simulink model "EX005_FCHEVwithCooling"  (R2023a)
settings: Solver=ode23tb  StartTime=0.0  StopTime=20e3  MaxStep=1e-1  RelTol=1e-4
libraries: component_lib x35, slpidlib x3, simulink x1
settings Model: Creator=maxjo65  LastModifiedBy=maxjo
settings OptimizationCC: ReuseModelBlockBuffer=off
settings DebuggingCC: UnconnectedInputMsg=warning  UnconnectedOutputMsg=warning  UnconnectedLineMsg=warning
settings ModelReferenceCC: EnableRefExpFcnMdlSchedulingChecks=on
settings RTWCC: DLArmComputeVersion=19.05

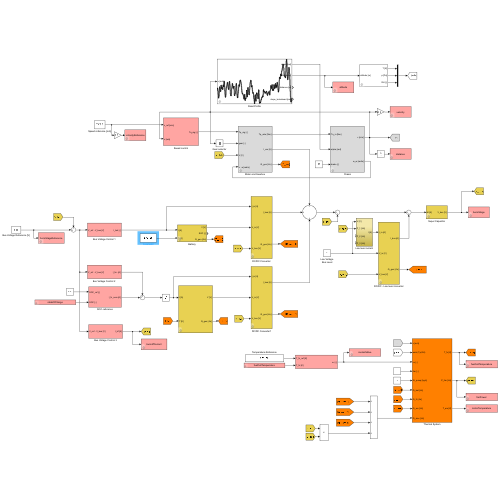
[thumbnail: Simulink's stored preview of the top-level diagram]
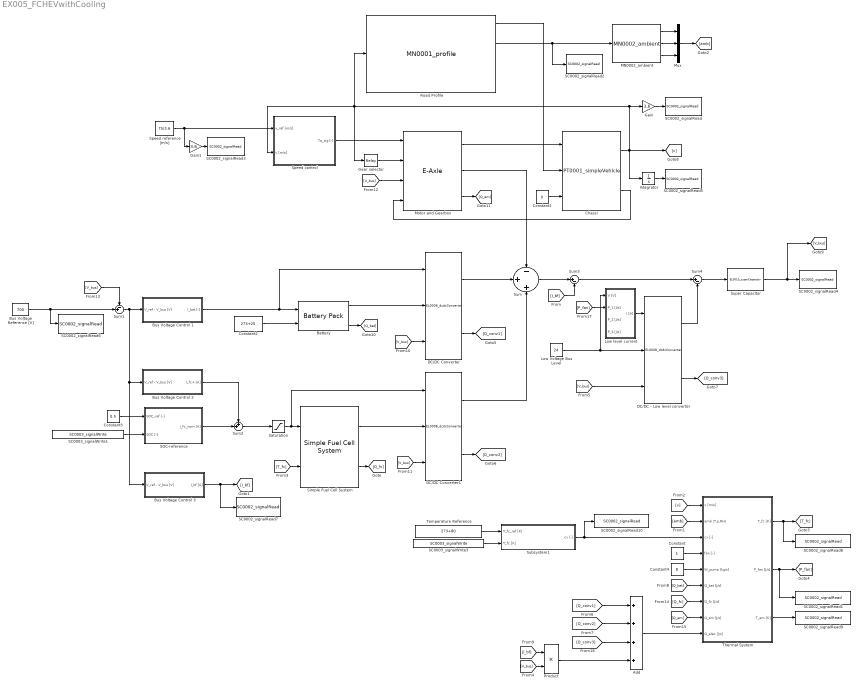
== system EX005_FCHEVwithCooling ==
  Add : Sum  Inputs=++++
  Battery : component_lib/Battery Pack  SOC_0=0.5  Nx=120  Ny=180
  Bus Voltage Control 1 : Subsystem
  "Bus Voltage Control 2 " : Subsystem
  Bus Voltage Control 3 : Subsystem
  Bus Voltage Reference [V] : Constant  Value=700
  Chassi : component_lib/Powertrain/PT0001_simpleVehicle  m=40e3  r_w=0.5  A_f=10  C_d=0.5  rho_air=1.225  c_r0=0.0060  c_r1=2.3e-7  gain=600  v0=75/3.6  x0=0
  Constant : Constant
  Constant1 : Constant  Value=0
  Constant2 : Constant  Value=273+25
  Constant3 : Constant  Value=0.5
  Constant4 : Constant  Value=8
  DC/DC - Low level converter : component_lib/Electrochemistry/EL0008_dcdcConverter  eta_up=0.99  eta_down=0.99
  DC/DC Converter : component_lib/Electrochemistry/EL0008_dcdcConverter  eta_up=0.99  eta_down=0.99
  DC/DC Converter1 : component_lib/Electrochemistry/EL0008_dcdcConverter  eta_up=0.99  eta_down=0.99
  Gain : Gain  Gain=3.6
  Gain1 : Gain  Gain=3.6
  Gear selector : Relay  OnSwitchValue=22  OffSwitchValue=21.5  OnOutputValue=4  OffOutputValue=3
  Integrator : Integrator
  Low Voltage Bus Level : Constant  Value=24
  Low level current : Subsystem
  MN0002_ambient : component_lib/Mission/MN0002_ambient  p_0=1.01e5  T_0=273 + 20  RH_0=0.05
  Motor and Gearbox : component_lib/E-Axle  n=3  V_nom=700
  Mux : Mux  Inputs=3
  Product : Product
  Road Profile : component_lib/Mission/MN0001_profile  profile=Sodertalje_Norrkoping.mat  x0=0  N_lookahead=100
  SC0002_signalRead : component_lib/Data & Control/SC0002_signalRead  SigName=velocity
  SC0002_signalRead1 : component_lib/Data & Control/SC0002_signalRead  SigName=fanPower
  SC0002_signalRead10 : component_lib/Data & Control/SC0002_signalRead  SigName=coolantValve
  SC0002_signalRead2 : component_lib/Data & Control/SC0002_signalRead  SigName=altitude
  SC0002_signalRead3 : component_lib/Data & Control/SC0002_signalRead  SigName=velocityReference
  SC0002_signalRead4 : component_lib/Data & Control/SC0002_signalRead  SigName=busVoltage
  SC0002_signalRead5 : component_lib/Data & Control/SC0002_signalRead  SigName=distance
  SC0002_signalRead6 : component_lib/Data & Control/SC0002_signalRead  SigName=busVoltageReference
  SC0002_signalRead7 : component_lib/Data & Control/SC0002_signalRead  SigName=burnoffCurrent
  SC0002_signalRead8 : component_lib/Data & Control/SC0002_signalRead  SigName=fuelCellTemperature
  SC0002_signalRead9 : component_lib/Data & Control/SC0002_signalRead  SigName=motorTemperature
  SC0003_signalWrite1 : component_lib/Data & Control/SC0003_signalWrite  SigName=stateOfCharge
  SC0003_signalWrite3 : component_lib/Data & Control/SC0003_signalWrite  SigName=fuelCellTemperature
  SOC-reference : Subsystem
  Saturation : Saturate  UpperLimit=600  LowerLimit=20
  Simple Fuel Cell System : component_lib/Simple Fuel Cell System  n_st=2  n=375
  Speed control : Subsystem
  Speed reference [m/s] : Constant  Value=75/3.6
  Subsystem1 : Subsystem
  Sum : Sum  Inputs=-++
  Sum1 : Sum  Inputs=-+|
  Sum2 : Sum  Inputs=++|
  Sum3 : Sum  Inputs=|+-
  Sum4 : Sum  Inputs=|+-
  Super Capacitor : component_lib/Electrochemistry/EL0010_superCapacitor  C=1  V_bus0=700
  Temperature Reference : Constant  Value=273+80
  Thermal System : Subsystem
  wires:
  Motor and Gearbox/1 -> Chassi/1
  Chassi/2 -> Motor and Gearbox/4
  Road Profile/1 -> Chassi/2
  Speed reference [m/s]/1 -> Gain1/1, Speed control/1(v_ref [m/s])
  Gear selector/1 -> Motor and Gearbox/2
  Integrator/1 -> SC0002_signalRead5/1
  Gain/1 -> SC0002_signalRead/1
  Road Profile/2 -> MN0002_ambient/1, SC0002_signalRead2/1
  Gain1/1 -> SC0002_signalRead3/1
  Super Capacitor/1 -> SC0002_signalRead4/1, [V_bus]
  Constant1/1 -> Chassi/3
  Battery/1 -> DC/DC Converter/2
  DC/DC Converter/1 -> Sum/2
  Motor and Gearbox/2 -> Sum/1
  Bus Voltage Control 1/1(I_bat [-]) -> Battery/1, DC/DC Converter/1
  DC/DC Converter1/1 -> Sum/3
  Bus Voltage Reference [V]/1 -> Sum1/2, SC0002_signalRead6/1
  Constant3/1 -> SOC-reference/1(SOC_ref [-])
  SC0003_signalWrite1/1 -> SOC-reference/2(SOC [-])
  Sum1/1 -> Bus Voltage Control 3/1(V_ref - V_bus [V]), "Bus Voltage Control 2 "/1(V_ref - V_bus [V]), Bus Voltage Control 1/1(V_ref - V_bus [V])
  "Bus Voltage Control 2 "/1(I_fc+ [A]) -> Sum2/1
  SOC-reference/1(I_fc_nom [A]) -> Sum2/2
  Sum/1 -> Sum3/1
  Bus Voltage Control 3/1(I_bf [A]) -> SC0002_signalRead7/1, [I_bf]
  [I_bf] -> Sum3/2
  MN0002_ambient/3 -> Mux/3
  MN0002_ambient/1 -> Mux/1
  MN0002_ambient/2 -> Mux/2
  Mux/1 -> [amb]
  Simple Fuel Cell System/1 -> DC/DC Converter1/2
  Saturation/1 -> Simple Fuel Cell System/1, DC/DC Converter1/1
  Sum3/1 -> Sum4/1
  Thermal System/2(P_fan [J/s]) -> [P_fan], SC0002_signalRead1/1
  Constant4/1 -> Thermal System/5(W_pump [kg/s])
  [Q_em] -> Thermal System/8(Q_em [J/s])
  Thermal System/1(T_fc [K]) -> [T_fc], SC0002_signalRead8/1
  [Q_bat] -> Thermal System/6(Q_bat [J/s])
  Subsystem1/1(cv [-]) -> Thermal System/3(cv [-]), SC0002_signalRead10/1
  [v] -> Thermal System/1(v [m/s])
  Constant/1 -> Thermal System/4(fan [-])
  Thermal System/3(T_em [K]) -> SC0002_signalRead9/1
  [Q_fc] -> Thermal System/7(Q_fc [J/s])
  [amb] -> Thermal System/2(amb (T,p,RH))
  Low Voltage Bus Level/1 -> DC/DC - Low level converter/2, Low level current/1(V [V])
  DC/DC - Low level converter/1 -> Sum4/2
  Sum4/1 -> Super Capacitor/1
  Add/1 -> Thermal System/9(Q_elec [J/s])
  [Q_conv1] -> Add/1
  [Q_conv2] -> Add/2
  [Q_conv3] -> Add/3
  DC/DC Converter/2 -> [Q_conv1]
  DC/DC Converter1/2 -> [Q_conv2]
  DC/DC - Low level converter/2 -> [Q_conv3]
  [V_bus] -> Motor and Gearbox/3
  [V_bus] -> Sum1/1
  Battery/3 -> [Q_bat]
  Simple Fuel Cell System/2 -> [Q_fc]
  [I_bf] -> Product/1
  [V_bus] -> Product/2
  Product/1 -> Add/4
  Motor and Gearbox/3 -> [Q_em]
  Temperature Reference/1 -> Subsystem1/1(T_fc_ref [K])
  Chassi/1 -> Integrator/1, [v], Gain/1, Road Profile/1, Speed control/2(v [m/s]), Gear selector/1
  SC0003_signalWrite3/1 -> Subsystem1/2(T_fc [K])
  [P_fan] -> Low level current/2(P_1 [J/s])
  [T_fc] -> Simple Fuel Cell System/2
  Speed control/1(Tq_sig [-]) -> Motor and Gearbox/1
  Sum2/1 -> Saturation/1
  [V_bus] -> DC/DC Converter/3
  [V_bus] -> DC/DC Converter1/3
  Constant2/1 -> Battery/2
  Low level current/1(I [A]) -> DC/DC - Low level converter/1
  [V_bus] -> DC/DC - Low level converter/3

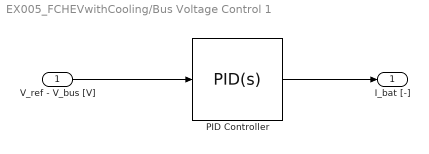
== system EX005_FCHEVwithCooling/Bus Voltage Control 1 ==
  V_ref - V_bus [V] : Inport
  PID Controller : slpidlib/PID Controller  Controller=PID  Form=Parallel  TimeDomain=Continuous-time  UseExternalTs=off  SampleTime=-1  IntegratorMethod=Forward Euler  FilterMethod=Forward Euler  ControllerParametersSource=internal  P=1e2  I=1  UseKiTs=off  D=0  N=100  UseFilter=on  TunerSelectOption=Transfer Function Based (PID Tuner App)  ZeroCross=off  InitialConditionSource=internal  InitialConditionForIntegrator=0  InitialConditionForFilter=0  DifferentiatorICPrevScaledInput=0  ExternalReset=none  TrackingMode=off  Kt=1  LimitOutput=on  SatLimitsSource=internal  UpperSaturationLimit=350  LowerSaturationLimit=-350  LinearizeAsGain=on  AntiWindupMode=clamping  Kb=1  LimitIntegrator=off  UpperIntegratorSaturationLimit=inf  LowerIntegratorSaturationLimit=-inf  POutMin=[]  POutMax=[]  IOutMin=[]  IOutMax=[]  DOutMin=[]  DOutMax=[]  NOutMin=[]  NOutMax=[]  SumOutMin=[]  SumOutMax=[]  SaturationOutMin=[]  SaturationOutMax=[]  PParamMin=[]  PParamMax=[]  IParamMin=[]  IParamMax=[]  DParamMin=[]  DParamMax=[]  NParamMin=[]  NParamMax=[]  KbParamMin=[]  KbParamMax=[]  KtParamMin=[]  KtParamMax=[]  KbOutMin=[]  KbOutMax=[]  KtOutMin=[]  KtOutMax=[]  IntegratorOutMin=[]  IntegratorOutMax=[]  FilterOutMin=[]  FilterOutMax=[]  SumI1OutMin=[]  SumI1OutMax=[]  SumI2OutMin=[]  SumI2OutMax=[]  SumI3OutMin=[]  SumI3OutMax=[]  SumI4OutMin=[]  SumI4OutMax=[]  SumDOutMin=[]  SumDOutMax=[]  DifferentiatorOutMin=[]  DifferentiatorOutMax=[]  FilterDiffOutCoefMin=[]  FilterDiffOutCoefMax=[]  ReciprocalOutMin=[]  ReciprocalOutMax=[]  SumDenOutMin=[]  SumDenOutMax=[]  SumNumOutMin=[]  SumNumOutMax=[]  DivideOutMin=[]  DivideOutMax=[]  UdiffTsProdOutMin=[]  UdiffTsProdOutMax=[]  NTsProdOutMin=[]  NTsProdOutMax=[]  UintegralTsProdOutMin=[]  UintegralTsProdOutMax=[]  UngainTsProdOutMin=[]  UngainTsProdOutMax=[]  ClampingZeroOutDataTypeStr=Inherit: Inherit via back propagation  ClampingZeroOutMin=[]  ClampingZeroOutMax=[]  FilterDenConstantOutDataTypeStr=Inherit: Inherit via back propagation  FilterDenConstantOutMin=[]  FilterDenConstantOutMax=[]  PCopyOutDataTypeStr=Inherit: Inherit via back propagation  PCopyOutMin=[]  PCopyOutMax=[]  NCopyOutDataTypeStr=Inherit: Inherit via back propagation  NCopyOutMin=[]  NCopyOutMax=[]  IntegratorContinuousStateAttributes=''  IntegratorStateMustResolveToSignalObject=off  IntegratorRTWStateStorageClass=Auto  FilterContinuousStateAttributes=''  FilterStateMustResolveToSignalObject=off  FilterRTWStateStorageClass=Auto  ParallelPVariant=InternalParameters  IdealPVariant=Disabled  IVariant=InternalParameters  DVariant=InternalParameters  IntegratorVariant=Continuous  SatVariant=Enabled  AWVariant=ContClampingParallel  PCopyVariant=Disabled  TRVariant=Disabled  FdbkBlocksVariant=Forward  IdealPFdbkVariant=Disabled  SatFdbkVariant=Disabled  DerivativeFilterVariant=ContFilter  NVariant=InternalParameters  NCopyVariant=Disabled  FilterICVariant=InternalICsFilter  IntegratorICVariant=InternalICs  ExternalResetVariant=Disabled  TRSumVariant=Passthrough  SumFdbkVariant=Disabled  SumVariant=Sum_PID  TsampFilterVariant=InternalTs  TsampNgainVariant=Passthrough  TsampIntegralVariant=Disabled_SignalSpec  ExternalSaturationOutDataTypeStr=Inherit: Same as second input
  I_bat [-] : Outport
  wires:
  PID Controller/1 -> I_bat [-]/1
  V_ref - V_bus [V]/1 -> PID Controller/1

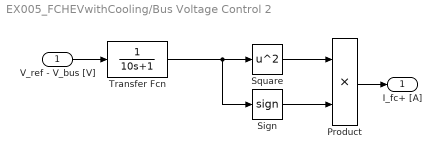
== system EX005_FCHEVwithCooling/Bus Voltage Control 2  ==
  V_ref - V_bus [V] : Inport
  Product : Product
  Sign : Signum
  Square : Math  Operator=square
  Transfer Fcn : TransferFcn  Denominator=[10 1]
  I_fc+ [A] : Outport
  wires:
  Sign/1 -> Product/2
  Transfer Fcn/1 -> Sign/1, Square/1
  Square/1 -> Product/1
  V_ref - V_bus [V]/1 -> Transfer Fcn/1
  Product/1 -> I_fc+ [A]/1

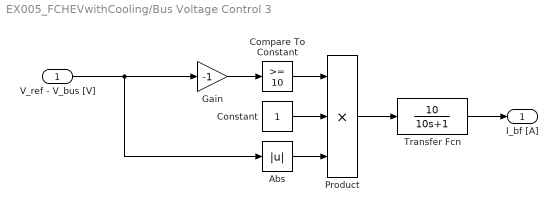
== system EX005_FCHEVwithCooling/Bus Voltage Control 3 ==
  V_ref - V_bus [V] : Inport
  Abs : Abs  SaturateOnIntegerOverflow=off
  Compare To Constant : simulink/Logic and Bit Operations/Compare To Constant  relop=>=  const=10  OutDataTypeStr=boolean
  Constant : Constant
  Gain : Gain  Gain=-1
  Product : Product  Inputs=3
  Transfer Fcn : TransferFcn  Numerator=[10]  Denominator=[10 1]
  I_bf [A] : Outport
  wires:
  Gain/1 -> Compare To Constant/1
  Transfer Fcn/1 -> I_bf [A]/1
  Compare To Constant/1 -> Product/1
  Product/1 -> Transfer Fcn/1
  V_ref - V_bus [V]/1 -> Abs/1, Gain/1
  Abs/1 -> Product/3
  Constant/1 -> Product/2

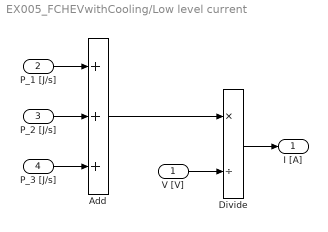
== system EX005_FCHEVwithCooling/Low level current ==
  V [V] : Inport
  P_1 [J/s] : Inport  Port=2
  P_2 [J/s] : Inport  Port=3
  P_3 [J/s] : Inport  Port=4
  Add : Sum  Inputs=+++
  Divide : Product  Inputs=*/
  I [A] : Outport
  wires:
  Add/1 -> Divide/1
  P_1 [J/s]/1 -> Add/1
  V [V]/1 -> Divide/2
  P_3 [J/s]/1 -> Add/3
  P_2 [J/s]/1 -> Add/2
  Divide/1 -> I [A]/1

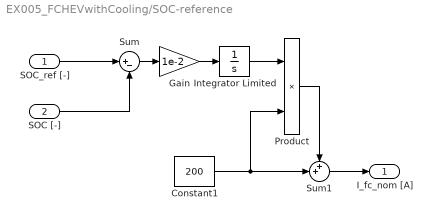
== system EX005_FCHEVwithCooling/SOC-reference ==
  SOC_ref [-] : Inport
  SOC [-] : Inport  Port=2
  Constant1 : Constant  Value=200
  Gain : Gain  Gain=1e-2
  Integrator Limited : Integrator  LimitOutput=on  UpperSaturationLimit=1  LowerSaturationLimit=-1
  Product : Product
  Sum : Sum  Inputs=|+-
  Sum1 : Sum  Inputs=++|
  I_fc_nom [A] : Outport
  wires:
  Product/1 -> Sum1/1
  Integrator Limited/1 -> Product/1
  Sum1/1 -> I_fc_nom [A]/1
  Constant1/1 -> Sum1/2, Product/2
  Sum/1 -> Gain/1
  SOC [-]/1 -> Sum/2
  Gain/1 -> Integrator Limited/1
  SOC_ref [-]/1 -> Sum/1

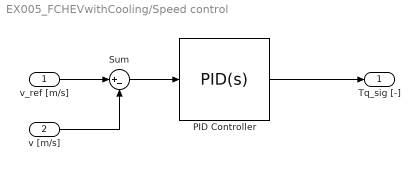
== system EX005_FCHEVwithCooling/Speed control ==
  v_ref [m/s] : Inport
  v [m/s] : Inport  Port=2
  PID Controller : slpidlib/PID Controller  Controller=PID  Form=Parallel  TimeDomain=Continuous-time  UseExternalTs=off  SampleTime=-1  IntegratorMethod=Forward Euler  FilterMethod=Forward Euler  ControllerParametersSource=internal  P=10  I=1e-1  UseKiTs=off  D=0  N=100  UseFilter=on  TunerSelectOption=Transfer Function Based (PID Tuner App)  ZeroCross=off  InitialConditionSource=internal  InitialConditionForIntegrator=0  InitialConditionForFilter=0  DifferentiatorICPrevScaledInput=0  ExternalReset=none  TrackingMode=off  Kt=1  LimitOutput=on  SatLimitsSource=internal  UpperSaturationLimit=1  LowerSaturationLimit=-1  LinearizeAsGain=on  AntiWindupMode=clamping  Kb=1  LimitIntegrator=off  UpperIntegratorSaturationLimit=inf  LowerIntegratorSaturationLimit=-inf  POutMin=[]  POutMax=[]  IOutMin=[]  IOutMax=[]  DOutMin=[]  DOutMax=[]  NOutMin=[]  NOutMax=[]  SumOutMin=[]  SumOutMax=[]  SaturationOutMin=[]  SaturationOutMax=[]  PParamMin=[]  PParamMax=[]  IParamMin=[]  IParamMax=[]  DParamMin=[]  DParamMax=[]  NParamMin=[]  NParamMax=[]  KbParamMin=[]  KbParamMax=[]  KtParamMin=[]  KtParamMax=[]  KbOutMin=[]  KbOutMax=[]  KtOutMin=[]  KtOutMax=[]  IntegratorOutMin=[]  IntegratorOutMax=[]  FilterOutMin=[]  FilterOutMax=[]  SumI1OutMin=[]  SumI1OutMax=[]  SumI2OutMin=[]  SumI2OutMax=[]  SumI3OutMin=[]  SumI3OutMax=[]  SumI4OutMin=[]  SumI4OutMax=[]  SumDOutMin=[]  SumDOutMax=[]  DifferentiatorOutMin=[]  DifferentiatorOutMax=[]  FilterDiffOutCoefMin=[]  FilterDiffOutCoefMax=[]  ReciprocalOutMin=[]  ReciprocalOutMax=[]  SumDenOutMin=[]  SumDenOutMax=[]  SumNumOutMin=[]  SumNumOutMax=[]  DivideOutMin=[]  DivideOutMax=[]  UdiffTsProdOutMin=[]  UdiffTsProdOutMax=[]  NTsProdOutMin=[]  NTsProdOutMax=[]  UintegralTsProdOutMin=[]  UintegralTsProdOutMax=[]  UngainTsProdOutMin=[]  UngainTsProdOutMax=[]  ClampingZeroOutDataTypeStr=Inherit: Inherit via back propagation  ClampingZeroOutMin=[]  ClampingZeroOutMax=[]  FilterDenConstantOutDataTypeStr=Inherit: Inherit via back propagation  FilterDenConstantOutMin=[]  FilterDenConstantOutMax=[]  PCopyOutDataTypeStr=Inherit: Inherit via back propagation  PCopyOutMin=[]  PCopyOutMax=[]  NCopyOutDataTypeStr=Inherit: Inherit via back propagation  NCopyOutMin=[]  NCopyOutMax=[]  IntegratorContinuousStateAttributes=''  IntegratorStateMustResolveToSignalObject=off  IntegratorRTWStateStorageClass=Auto  FilterContinuousStateAttributes=''  FilterStateMustResolveToSignalObject=off  FilterRTWStateStorageClass=Auto  ParallelPVariant=InternalParameters  IdealPVariant=Disabled  IVariant=InternalParameters  DVariant=InternalParameters  IntegratorVariant=Continuous  SatVariant=Enabled  AWVariant=ContClampingParallel  PCopyVariant=Disabled  TRVariant=Disabled  FdbkBlocksVariant=Forward  IdealPFdbkVariant=Disabled  SatFdbkVariant=Disabled  DerivativeFilterVariant=ContFilter  NVariant=InternalParameters  NCopyVariant=Disabled  FilterICVariant=InternalICsFilter  IntegratorICVariant=InternalICs  ExternalResetVariant=Disabled  TRSumVariant=Passthrough  SumFdbkVariant=Disabled  SumVariant=Sum_PID  TsampFilterVariant=InternalTs  TsampNgainVariant=Passthrough  TsampIntegralVariant=Disabled_SignalSpec  ExternalSaturationOutDataTypeStr=Inherit: Same as second input
  Sum : Sum  Inputs=|+-
  Tq_sig [-] : Outport
  wires:
  PID Controller/1 -> Tq_sig [-]/1
  Sum/1 -> PID Controller/1
  v_ref [m/s]/1 -> Sum/1
  v [m/s]/1 -> Sum/2

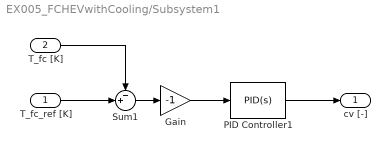
== system EX005_FCHEVwithCooling/Subsystem1 ==
  T_fc_ref [K] : Inport
  T_fc [K] : Inport  Port=2
  Gain : Gain  Gain=-1
  PID Controller1 : slpidlib/PID Controller  Controller=PID  Form=Parallel  TimeDomain=Continuous-time  UseExternalTs=off  SampleTime=-1  IntegratorMethod=Forward Euler  FilterMethod=Forward Euler  ControllerParametersSource=internal  P=1e-1  I=1e-2  UseKiTs=off  D=0  N=100  UseFilter=on  TunerSelectOption=Transfer Function Based (PID Tuner App)  ZeroCross=off  InitialConditionSource=internal  InitialConditionForIntegrator=0.5  InitialConditionForFilter=0.5  DifferentiatorICPrevScaledInput=0  ExternalReset=none  TrackingMode=off  Kt=1  LimitOutput=on  SatLimitsSource=internal  UpperSaturationLimit=0.95  LowerSaturationLimit=0.05  LinearizeAsGain=on  AntiWindupMode=clamping  Kb=1  LimitIntegrator=off  UpperIntegratorSaturationLimit=inf  LowerIntegratorSaturationLimit=-inf  POutMin=[]  POutMax=[]  IOutMin=[]  IOutMax=[]  DOutMin=[]  DOutMax=[]  NOutMin=[]  NOutMax=[]  SumOutMin=[]  SumOutMax=[]  SaturationOutMin=[]  SaturationOutMax=[]  PParamMin=[]  PParamMax=[]  IParamMin=[]  IParamMax=[]  DParamMin=[]  DParamMax=[]  NParamMin=[]  NParamMax=[]  KbParamMin=[]  KbParamMax=[]  KtParamMin=[]  KtParamMax=[]  KbOutMin=[]  KbOutMax=[]  KtOutMin=[]  KtOutMax=[]  IntegratorOutMin=[]  IntegratorOutMax=[]  FilterOutMin=[]  FilterOutMax=[]  SumI1OutMin=[]  SumI1OutMax=[]  SumI2OutMin=[]  SumI2OutMax=[]  SumI3OutMin=[]  SumI3OutMax=[]  SumI4OutMin=[]  SumI4OutMax=[]  SumDOutMin=[]  SumDOutMax=[]  DifferentiatorOutMin=[]  DifferentiatorOutMax=[]  FilterDiffOutCoefMin=[]  FilterDiffOutCoefMax=[]  ReciprocalOutMin=[]  ReciprocalOutMax=[]  SumDenOutMin=[]  SumDenOutMax=[]  SumNumOutMin=[]  SumNumOutMax=[]  DivideOutMin=[]  DivideOutMax=[]  UdiffTsProdOutMin=[]  UdiffTsProdOutMax=[]  NTsProdOutMin=[]  NTsProdOutMax=[]  UintegralTsProdOutMin=[]  UintegralTsProdOutMax=[]  UngainTsProdOutMin=[]  UngainTsProdOutMax=[]  ClampingZeroOutDataTypeStr=Inherit: Inherit via back propagation  ClampingZeroOutMin=[]  ClampingZeroOutMax=[]  FilterDenConstantOutDataTypeStr=Inherit: Inherit via back propagation  FilterDenConstantOutMin=[]  FilterDenConstantOutMax=[]  PCopyOutDataTypeStr=Inherit: Inherit via back propagation  PCopyOutMin=[]  PCopyOutMax=[]  NCopyOutDataTypeStr=Inherit: Inherit via back propagation  NCopyOutMin=[]  NCopyOutMax=[]  IntegratorContinuousStateAttributes=''  IntegratorStateMustResolveToSignalObject=off  IntegratorRTWStateStorageClass=Auto  FilterContinuousStateAttributes=''  FilterStateMustResolveToSignalObject=off  FilterRTWStateStorageClass=Auto  ParallelPVariant=InternalParameters  IdealPVariant=Disabled  IVariant=InternalParameters  DVariant=InternalParameters  IntegratorVariant=Continuous  SatVariant=Enabled  AWVariant=ContClampingParallel  PCopyVariant=Disabled  TRVariant=Disabled  FdbkBlocksVariant=Forward  IdealPFdbkVariant=Disabled  SatFdbkVariant=Disabled  DerivativeFilterVariant=ContFilter  NVariant=InternalParameters  NCopyVariant=Disabled  FilterICVariant=InternalICsFilter  IntegratorICVariant=InternalICs  ExternalResetVariant=Disabled  TRSumVariant=Passthrough  SumFdbkVariant=Disabled  SumVariant=Sum_PID  TsampFilterVariant=InternalTs  TsampNgainVariant=Passthrough  TsampIntegralVariant=Disabled_SignalSpec  ExternalSaturationOutDataTypeStr=Inherit: Same as second input
  Sum1 : Sum  Inputs=-+|
  cv [-] : Outport
  wires:
  T_fc [K]/1 -> Sum1/1
  Gain/1 -> PID Controller1/1
  Sum1/1 -> Gain/1
  PID Controller1/1 -> cv [-]/1
  T_fc_ref [K]/1 -> Sum1/2

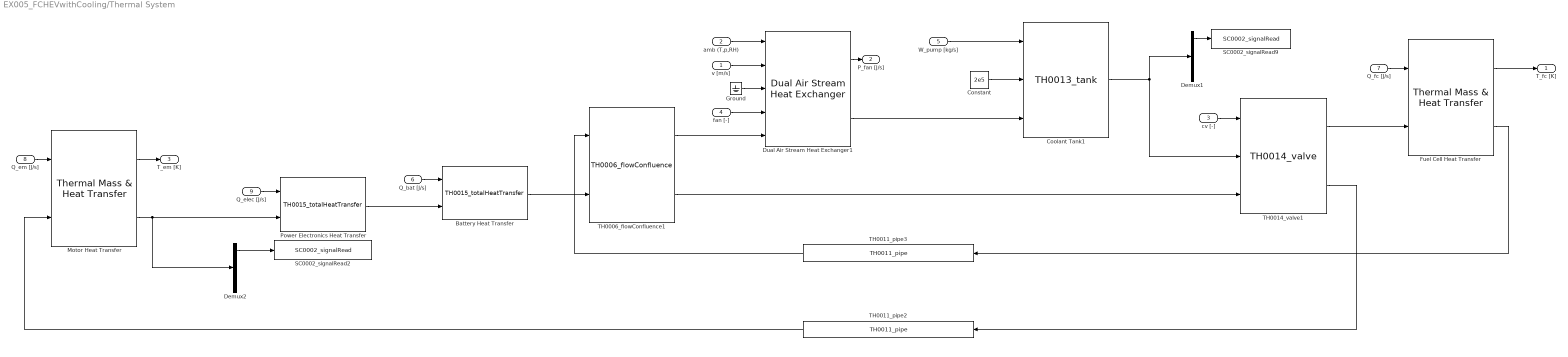
== system EX005_FCHEVwithCooling/Thermal System ==
  v [m/s] : Inport
  amb (T,p,RH) : Inport  Port=2
  cv [-] : Inport  Port=3
  fan [-] : Inport  Port=4
  W_pump [kg/s] : Inport  Port=5
  Q_bat [J/s] : Inport  Port=6
  Q_fc [J/s] : Inport  Port=7
  Q_em [J/s] : Inport  Port=8
  Q_elec [J/s] : Inport  Port=9
  Battery Heat Transfer : component_lib/Thermal Systems/TH0015_totalHeatTransfer  T_max=273+100  T_min=273
  Constant : Constant  Value=2e5
  Coolant Tank1 : component_lib/Thermal Systems/TH0013_tank  V=5e-3  T0=273.15 + 80
  Demux1 : Demux  Outputs=3
  Demux2 : Demux  Outputs=3
  Dual Air Stream Heat Exchanger1 : component_lib/Dual Air Stream Heat Exchanger  HtH=1.1  StS=0.95
  Fuel Cell Heat Transfer : component_lib/Thermal Mass & Heat Transfer  n=375*2*10  d=2e-3  L=50e-2  m=72  cp=420  T_0=273 + 80
  Ground : Ground
  Motor Heat Transfer : component_lib/Thermal Mass & Heat Transfer  n=100*3  d=5e-3  L=30e-2  m=200  cp=420  T_0=273 + 20
  Power Electronics Heat Transfer : component_lib/Thermal Systems/TH0015_totalHeatTransfer  T_max=273+100  T_min=273
  SC0002_signalRead2 : component_lib/Data & Control/SC0002_signalRead  SigName=powerElectronicsTemperature
  SC0002_signalRead9 : component_lib/Data & Control/SC0002_signalRead  SigName=coolantTemperature
  TH0006_flowConfluence1 : component_lib/Thermal Systems/TH0006_flowConfluence  gain=0.01
  TH0011_pipe2 : component_lib/Thermal Systems/TH0011_pipe  d=3e-2  L=2  e=0.006e-3  T_0=273 + 20
  TH0011_pipe3 : component_lib/Thermal Systems/TH0011_pipe  d=3e-2  L=2  e=0.006e-3  T_0=273 + 20
  TH0014_valve1 : component_lib/Thermal Systems/TH0014_valve  d=10e-2  dr=5e-2  C_d=0.9
  T_fc [K] : Outport
  P_fan [J/s] : Outport  Port=2
  T_em [K] : Outport  Port=3
  wires:
  Demux2/1 -> SC0002_signalRead2/1
  TH0014_valve1/2 -> TH0011_pipe2/1
  Power Electronics Heat Transfer/1 -> Battery Heat Transfer/2
  cv [-]/1 -> TH0014_valve1/1
  TH0006_flowConfluence1/1 -> Dual Air Stream Heat Exchanger1/5
  Coolant Tank1/1 -> Demux1/1, TH0014_valve1/2
  TH0006_flowConfluence1/2 -> TH0014_valve1/3
  amb (T,p,RH)/1 -> Dual Air Stream Heat Exchanger1/1
  Battery Heat Transfer/1 -> TH0006_flowConfluence1/2
  Ground/1 -> Dual Air Stream Heat Exchanger1/3
  fan [-]/1 -> Dual Air Stream Heat Exchanger1/4
  Motor Heat Transfer/2 -> Power Electronics Heat Transfer/2, Demux2/1
  Fuel Cell Heat Transfer/2 -> TH0011_pipe3/1
  TH0014_valve1/1 -> Fuel Cell Heat Transfer/2
  Q_elec [J/s]/1 -> Power Electronics Heat Transfer/1
  v [m/s]/1 -> Dual Air Stream Heat Exchanger1/2
  TH0011_pipe3/1 -> TH0006_flowConfluence1/1
  TH0011_pipe2/1 -> Motor Heat Transfer/2
  Q_fc [J/s]/1 -> Fuel Cell Heat Transfer/1
  Q_em [J/s]/1 -> Motor Heat Transfer/1
  Fuel Cell Heat Transfer/1 -> T_fc [K]/1
  Dual Air Stream Heat Exchanger1/1 -> P_fan [J/s]/1
  Motor Heat Transfer/1 -> T_em [K]/1
  Q_bat [J/s]/1 -> Battery Heat Transfer/1
  Demux1/1 -> SC0002_signalRead9/1
  Dual Air Stream Heat Exchanger1/2 -> Coolant Tank1/3
  W_pump [kg/s]/1 -> Coolant Tank1/1
  Constant/1 -> Coolant Tank1/2
